simulink model "binocularRivalry"  (R2024b)
settings: Solver=ode3  StartTime=0.0  StopTime=20.0  RelTol=1e-3
values from neighbouring files (symbols this model uses):
  a = x(7)    [binocularRivalryModel.m]    (also in main.m = 3.4)
  epsilon = x(9)    [binocularRivalryModel.m]    (also in main.m = 0)
  g = x(10)    [binocularRivalryModel.m]    (also in main.m = 3)
  L = x(5)    [binocularRivalryModel.m]    (also in main.m = 1)
  m = x(8)    [binocularRivalryModel.m]    (also in main.m = 1)
  R = x(6)    [binocularRivalryModel.m]    (also in main.m = R_values(i))
  tau = x(11)    [binocularRivalryModel.m]    (also in main.m = 0.015)
  tau_H = x(12)    [binocularRivalryModel.m]    (also in main.m = 1)
  x0 = [0, 0, 0, 0]    [main.m]
settings Model: Creator=marioroca  LastModifiedBy=marioroca

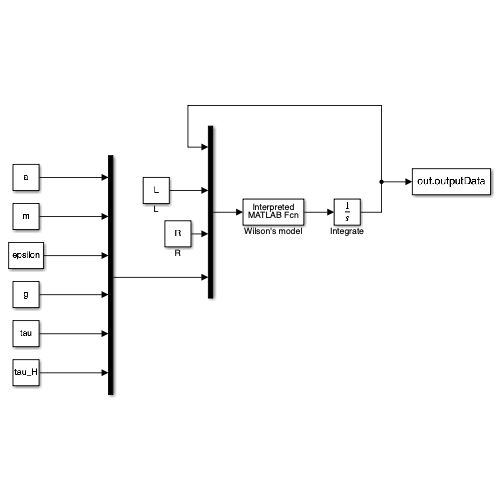
[thumbnail: Simulink's stored preview of the top-level diagram]
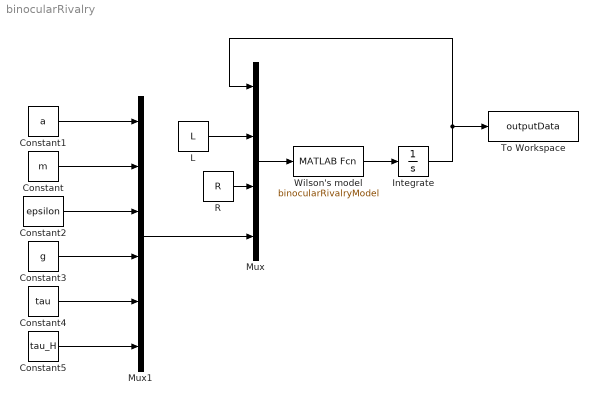
== system binocularRivalry ==
  Constant : Constant  Value=m
  Constant1 : Constant  Value=a
  Constant2 : Constant  Value=epsilon
  Constant3 : Constant  Value=g
  Constant4 : Constant  Value=tau
  Constant5 : Constant  Value=tau_H
  Integrate : Integrator  InitialCondition=x0
  L : Constant  Value=L
  Mux : Mux
  Mux1 : Mux  Inputs=6
  R : Constant  Value=R
  To Workspace : ToWorkspace  VariableName=outputData  SaveFormat=Timeseries  SampleTime=-1
  Wilson's model : MATLABFcn  MATLABFcn=binocularRivalryModel
  wires:
  L/1 -> Mux/2
  R/1 -> Mux/3
  Mux/1 -> Wilson's model/1
  Wilson's model/1 -> Integrate/1
  Integrate/1 -> To Workspace/1, Mux/1
  Constant2/1 -> Mux1/3
  Mux1/1 -> Mux/4
  Constant1/1 -> Mux1/1
  Constant/1 -> Mux1/2
  Constant3/1 -> Mux1/4
  Constant4/1 -> Mux1/5
  Constant5/1 -> Mux1/6
